simulink model "power_syncmachine"  (Simulink 6.0)
settings: Solver=ode15s  SolverMode=SingleTasking  StartTime=0.0  StopTime=3  FixedStep=300e-6  RelTol=1e-3
undefined symbols (not defined in the file or in its folder): gcbh, powericon
libraries: powerlib x5
settings Model: Creator=patrice  LastModifiedBy=batserve  ExtModeTrigMode=oneshot  ExtModeArmWhenConnect=off  ExtModeAutoUpdateStatusClock=off
settings DataIOCC: InitialState=xFinal  LimitDataPoints=off  SaveOutput=off  TimeSaveName=t  SignalLoggingName=sigsOut
settings OptimizationCC: BlockReduction=off  BooleanDataType=off
settings DebuggingCC: SolverPrmCheckMsg=none  UnconnectedInputMsg=none  UnconnectedOutputMsg=none
settings HardwareCC: TargetUnknown=on
settings RTWCC: TemplateMakefile=grt_unix.tmf

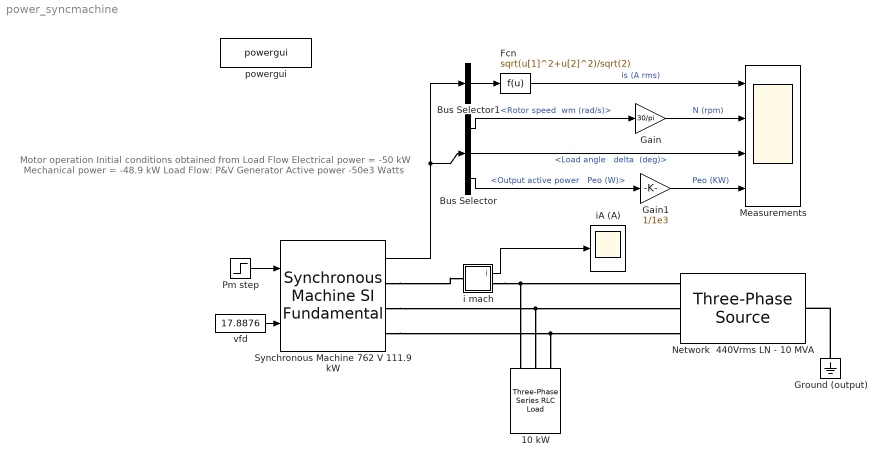
== system power_syncmachine ==
  note: Motor operation
      | Initial  conditions obtained from Load Flow
      | Electrical power = -50 kW
      | Mechanical power = -48.9 kW
      |
      | Load Flow:
      | P&V Generator
      | Active power -50e3 Watts
  10 kW : powerlib/Elements/Three-Phase Series RLC Load  Orientation=down  PhysicalDomain=powersysdomain  SubClassName=unknown  LeftPortType=p1  RightPortType=p1  LConnTagsString=A|B|C  Configuration=Y (grounded)  NominalVoltage=762  NominalFrequency=60  ActivePower=10e3  InductivePower=0  CapacitivePower=0  Measurements=None
  Bus Selector : BusSelector  DialogController=Simulink.DDGSource_Bus  OutputSignals="Mechanical.Rotor speed  wm (rad/s),Load angle   delta  (deg),Output active power   Peo (W)"
  Bus Selector1 : BusSelector  DialogController=Simulink.DDGSource_Bus  OutputSignals="dq0 components.Stator current  iq (A),dq0 components.Stator current  id (A)"  MuxedOutput=on
  Fcn : Fcn  Expr=sqrt(u[1]^2+u[2]^2)/sqrt(2)
  Gain : Gain  Gain=30/pi  SaturateOnIntegerOverflow=on
  Gain1 : Gain  Gain=1/1e3  SaturateOnIntegerOverflow=on
  Ground (output) : powerlib/Elements/Ground  Orientation=down  PhysicalDomain=powersysdomain  SubClassName=unknown  LeftPortType=p1  RightPortType=p1  LConnTagsString=a
  Measurements : Scope  NumInputPorts=4
      settings: TickLabels=on  TimeRange=1  YMin=37.5~1798.25~-26.5~-70  YMax=52.5~1800.25~-21~-50  SaveName=is2
  Network  440Vrms LN - 10 MVA : powerlib/Electrical Sources/Three-Phase Source  Orientation=left  Voltage=440*sqrt(3)  PhaseAngle=0  Frequency=60  InternalConnection=Yn  SpecifyImpedance=off  Resistance=762^2/10e6/10  Inductance=762^2/10e6/(2*pi*60)  ShortCircuitLevel=100e6  BaseVoltage=25e3  XRratio=7
  Pm step : Step  Time=0.1  Before=-48863  After=-60000  SampleTime=0
  Synchronous Machine 762 V 111.9 kW : powerlib/Machines/Synchronous Machine SI Fundamental  PresetModel=No  ShowDetailedParameters=on  RotorType=Salient-pole  NominalParameters="[ 111.9e3 440*sqrt(3)  60  0]"  Stator=[ .26 1.14e-3 13.7e-3 11.0e-3 ]  Field=[ 0.13 2.1e-3 ]  Dampers2=[ 1 2 3 4 5 6 ]  Dampers1=[ 0.0224 1.4e-3 0.02 1e-3 ]  Mechanical=[ 24.9 0 2 ]  InitialConditions=[0 -111.483 53.9768 53.9768 53.9768 -173.297 66.7033 -53.2967 17.8876]  SetSaturation=off  Saturation=[]  DisplayVfd=off  Units=1  LoadFlowParameters=[1,0,0,0,0]
      settings: AttributesFormatString=\n
  i mach : Subsystem  Tag=PoWeRsYsTeMmEaSuReMeNt  AncestorBlock=powerlib/Measurements/Current Measurement  LoadFcn=powericon('psbloadfunction',gcbh,'Measurement Block','');  InitFcn=powericon('psbloadfunction',gcbh,'InitFcnOfSPSBlocks','Measurement Block');  mask(Current Measurement){PhasorSimulation=off, OutputType=Magnitude, PSBequivalent=0}
      mask prompts: PhasorSimulation "Phasor simulation"; OutputType "Output signal :"; PSBequivalent "Equivalent circuit"
      mask help: Ideal current measurement.
      mask init:
      | switch OutputType
      | case 1
      |     OutputSelection = 1;
      |     NormalMode = 2;
      |     PhasorMode = 1;
      | case 2
      |     OutputSelection =[2,3];
      |     NormalMode = 3;
      |     PhasorMode = [1,2];
      | case 3
      |     OutputSelection =[4,5];
      |     NormalMode = 3;
      |     PhasorMode = [1,2];
      | case 4
      |     OutputSelection =[4];
      |     NormalMode = 2;
      |     PhasorMode = 1;
      | end
      | %
      | if PhasorSimulation
      |     SelectionMode = PhasorMode;
      | else
      |     SelectionMode = NormalMode;
      | end
      settings: AttributesFormatString=\n  CopyFcn=powericon('psbloadfunction',gcbh,'Measurement Block','VerifyPhasor');  PreSaveFcn=powericon('psbloadfunction',gcbh,'ModelCloseFcn','');  CloseFcn=powericon('psbloadfunction',gcbh,'CloseFcn','');
      mask Help: web(psbhelp);
      mask StyleString: checkbox,popup(Complex|Real-Imag|Magnitude-Angle|Magnitude),edit
  iA (A) : Scope
      settings: TickLabels=on  TimeRange=1  YMin=430  YMax=520  SaveName=is1  DataFormat=Array
  powergui : powerlib/powergui  Priority=2  Frange=logspace(0,3,50)  Ylog=off  Xlog=off  save=off  variable=ZData  ZoomFFT=on  StartTime=0.0  cycles=2  DisplayStyle=off  fundamental=60  FreqAxis=off  MaxFrequency=1000  frequencyindice=1  frequencyindicesteady=1  RmsSteady=1  display=off  Ts=0  methode=off  frequency=60  echomessages=off
  vfd : Constant  Value=17.8876
  wires:
  Fcn/1 -> Measurements/1  "is (A rms)"
  Bus Selector1/1 -> Fcn/1
  Gain/1 -> Measurements/2  "N (rpm)"
  Gain1/1 -> Measurements/4  "Peo (KW)"
  Synchronous Machine 762 V 111.9 kW/1 -> Bus Selector/1, Bus Selector1/1
  vfd/1 -> Synchronous Machine 762 V 111.9 kW/2
  Pm step/1 -> Synchronous Machine 762 V 111.9 kW/1
  i mach/1(i) -> iA (A)/1
  Bus Selector/3 -> Gain1/1  "<Output active power   Peo (W)>"
  Bus Selector/2 -> Measurements/3  "<Load angle   delta  (deg)>"
  Bus Selector/1 -> Gain/1  "<Rotor speed  wm (rad/s)>"
  connections:
  Synchronous Machine 762 V 111.9 kW/RConn1 -- i mach/LConn1
  Ground (output)/LConn1 -- Network  440Vrms LN - 10 MVA/LConn1
  Synchronous Machine 762 V 111.9 kW/RConn3 -- Network  440Vrms LN - 10 MVA/RConn3 -- 10 kW/LConn3
  Synchronous Machine 762 V 111.9 kW/RConn2 -- Network  440Vrms LN - 10 MVA/RConn2 -- 10 kW/LConn2
  i mach/RConn1 -- Network  440Vrms LN - 10 MVA/RConn1 -- 10 kW/LConn1

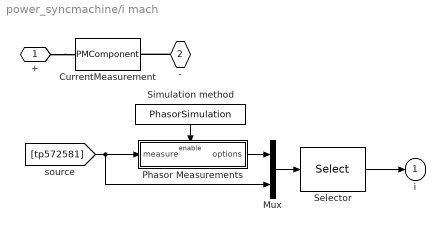
== system power_syncmachine/i mach ==
  CurrentMeasurement : PMComponent  PhysicalDomain=powersysdomain  LeftPortType=p1  RightPortType=p1  LConnTagsString=a  RConnTagsString=__new0
      mask Type: InnerPowersysBlock
  Mux : Mux  Inputs=2
  Phasor Measurements : Subsystem  TreatAsAtomicUnit=on
  Selector : Selector  Elements=SelectionMode  InputPortWidth=length(OutputSelection)+1
  Simulation method : Constant  Orientation=down  Value=PhasorSimulation
  + : PMIOPort  Port=1  Side=Left
  - : PMIOPort  Orientation=left  Port=2  Side=Right
  i : Outport  InitialOutput=0
  wires:
  Simulation method/1 -> Phasor Measurements/Enable
  Mux/1 -> Selector/1
  Phasor Measurements/1(options) -> Mux/1
  [tp572581] -> Mux/2, Phasor Measurements/1(measure)
  Selector/1 -> i/1
  connections:
  +/RConn1 -- CurrentMeasurement/LConn1
  -/RConn1 -- CurrentMeasurement/RConn1

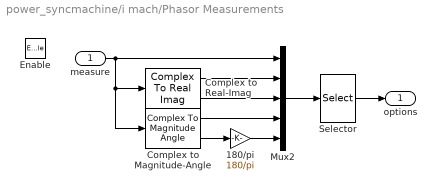
== system power_syncmachine/i mach/Phasor Measurements ==
  measure : Inport  Port=1  LatchInput=off
  Enable : EnablePort
  180/pi : Gain  Gain=180/pi  SaturateOnIntegerOverflow=on
  Complex to Magnitude-Angle : ComplexToMagnitudeAngle
  Complex to Real-Imag : ComplexToRealImag
  Mux2 : Mux  Inputs=5
  Selector : Selector  Elements=OutputSelection  InputPortWidth=5
  options : Outport  InitialOutput=0
  wires:
  Mux2/1 -> Selector/1
  measure/1 -> Complex to Magnitude-Angle/1, Complex to Real-Imag/1, Mux2/1
  Complex to Real-Imag/1 -> Mux2/2
  Complex to Real-Imag/2 -> Mux2/3
  Complex to Magnitude-Angle/1 -> Mux2/4
  Complex to Magnitude-Angle/2 -> 180/pi/1
  180/pi/1 -> Mux2/5
  Selector/1 -> options/1
